simulink model "stellaris_lp_adc"  (R2017a)
settings: Solver=FixedStepDiscrete  StartTime=0.0  StopTime=10.0  FixedStep=0.2  RelTol=1e-3
libraries: stellaris_lp_lib x15, simulink x1
settings Model: ExtModeTrigDuration=2  Creator=peselnikmg  LastModifiedBy=Nilim
settings DataIOCC: LimitDataPoints=on  SaveFormat=Array  SignalLoggingSaveFormat=ModelDataLogs  ReturnWorkspaceOutputs=on
settings OptimizationCC: UseDivisionForNetSlopeComputation=on  UseFloatMulNetSlope=on  UseSpecifiedMinMax=on  PassReuseOutputArgsAs=Individual arguments  ExpressionDepthLimit=2147483647  ZeroExternalMemoryAtStartup=off  ZeroInternalMemoryAtStartup=off  NoFixptDivByZeroProtection=on  EfficientFloat2IntCast=on  LifeSpan=inf  MaxStackSize=64  OptimizeBlockOrder=speed
settings DebuggingCC: ReadBeforeWriteMsg=DisableAll  WriteAfterWriteMsg=DisableAll  WriteAfterReadMsg=DisableAll  MultiTaskDSMMsg=none  IntegerOverflowMsg=error  ParameterTunabilityLossMsg=error  AssertControl=DisableAll  StateNameClashWarn=warning  NonBusSignalsTreatedAsBus=error  SFInvalidInputDataAccessInChartInitDiag=error  SFTransitionOutsideNaturalParentDiag=error  SFUnreachableExecutionPathDiag=error  SFUndirectedBroadcastEventsDiag=error  SFExecutionAtInitializationDiag=none  IntegerSaturationMsg=error
settings HardwareCC: ProdBitPerPointer=32  ProdBitPerSizeT=32  ProdBitPerPtrDiffT=32  ProdLargestAtomicInteger=Long  ProdLargestAtomicFloat=Double  ProdWordSize=32  ProdHWDeviceType=ARM Compatible->ARM Cortex
settings ModelReferenceCC: UpdateModelReferenceTargets=IfOutOfDate  PropagateSignalLabelsOutOfModel=off
settings SFSimCC: SFSimEcho=off  MATLABDynamicMemAlloc=off
settings RTWCC: SystemTargetFile=ert.tlc  HardwareBoard=Tiva TM4C123G Launchpad  TLCOptions=-aInlineSetEventsForThisBaseRateFcn=TLC_FALSE -aSuppressMultiTaskScheduler=TLC_FALSE -aRateBasedStepFcn=1  TemplateMakefile=ert_default_tmf  Description=Embedded Coder  GenerateReport=on  RTWVerbose=off  Toolchain=Texas Instruments Code Composer Studio (Tiva)  IncludeHyperlinkInReport=on  LaunchReport=on  GenerateTraceInfo=on  GenerateTraceReport=on  GenerateTraceReportSl=on  GenerateTraceReportSf=on  GenerateTraceReportEml=on
settings CodeAppCC: ForceParamTrailComments=on  IgnoreCustomStorageClasses=off  OperatorAnnotations=on  SimulinkDataObjDesc=on  SFDataObjDesc=on  MATLABFcnDesc=on  CustomSymbolStrType=$N$R$M  InsertBlockDesc=on  MATLABSourceComments=on  EnableCustomComments=on  ReqsInCode=on
settings ERTTargetCC: UtilityFuncGeneration=Shared location  CombineSignalStateStructs=on  SuppressErrorStatus=on  SupportNonFinite=off  ParenthesesLevel=Maximum  CastingMode=Standards  EnableSignedLeftShifts=off  EnableSignedRightShifts=off
settings ConfigComp: CovMetricSettings=dw  CovHtmlReporting=on  CovSaveCumulativeToWorkspaceVar=on  CovSaveSingleToWorkspaceVar=on  CovExternalEMLEnable=off

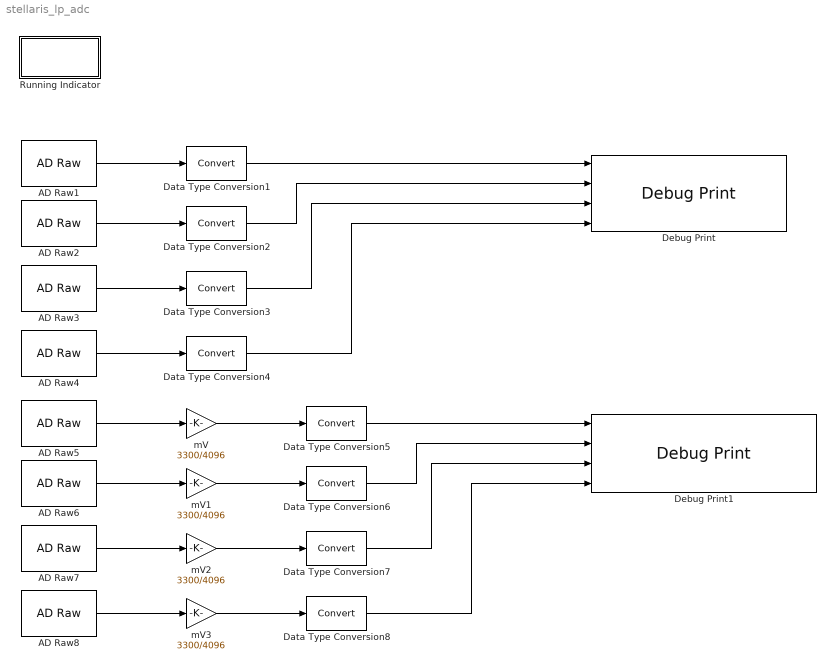
== system stellaris_lp_adc ==
  AD Raw1 : stellaris_lp_lib/ADC/AD Raw  ch="1   PE3"  sample_time=0.2
      settings: SourceProductName=Run on Stellaris LaunchPad
  AD Raw2 : stellaris_lp_lib/ADC/AD Raw  ch="2   PE2"  sample_time=0.2
      settings: SourceProductName=Run on Stellaris LaunchPad
  AD Raw3 : stellaris_lp_lib/ADC/AD Raw  ch="3   PE1"  sample_time=0.2
      settings: SourceProductName=Run on Stellaris LaunchPad
  AD Raw4 : stellaris_lp_lib/ADC/AD Raw  ch="4   PE0"  sample_time=0.2
      settings: SourceProductName=Run on Stellaris LaunchPad
  AD Raw5 : stellaris_lp_lib/ADC/AD Raw  ch="5   PE5"  sample_time=0.2
      settings: SourceProductName=Run on Stellaris LaunchPad
  AD Raw6 : stellaris_lp_lib/ADC/AD Raw  ch="6   PE4"  sample_time=0.2
      settings: SourceProductName=Run on Stellaris LaunchPad
  AD Raw7 : stellaris_lp_lib/ADC/AD Raw  ch="7   PB4"  sample_time=0.2
      settings: SourceProductName=Run on Stellaris LaunchPad
  AD Raw8 : stellaris_lp_lib/ADC/AD Raw  ch="8   PB5"  sample_time=0.2
      settings: SourceProductName=Run on Stellaris LaunchPad
  Data Type Conversion{1..8} (8 alike) : DataTypeConversion
  Debug Print : stellaris_lp_lib/Debug/Debug Print  fmt="'AD 1-4  = %d, %d, %d, %d'"  sample_time=-1
      settings: SourceProductName=Run on Stellaris LaunchPad
  Debug Print1 : stellaris_lp_lib/Debug/Debug Print  fmt="'AD 5-8  = %d, %d, %d, %d (unit mV)'"  sample_time=-1
      settings: SourceProductName=Run on Stellaris LaunchPad
  Running Indicator : Subsystem
  mV{,1..3} (4 alike) : Gain  Gain=3300/4096
  wires:
  Data Type Conversion1/1 -> Debug Print/1
  AD Raw1/1 -> Data Type Conversion1/1
  AD Raw2/1 -> Data Type Conversion2/1
  AD Raw3/1 -> Data Type Conversion3/1
  AD Raw4/1 -> Data Type Conversion4/1
  Data Type Conversion2/1 -> Debug Print/2
  Data Type Conversion3/1 -> Debug Print/3
  Data Type Conversion4/1 -> Debug Print/4
  Data Type Conversion5/1 -> Debug Print1/1
  AD Raw5/1 -> mV/1
  AD Raw6/1 -> mV1/1
  AD Raw7/1 -> mV2/1
  AD Raw8/1 -> mV3/1
  Data Type Conversion6/1 -> Debug Print1/2
  Data Type Conversion7/1 -> Debug Print1/3
  Data Type Conversion8/1 -> Debug Print1/4
  mV/1 -> Data Type Conversion5/1
  mV1/1 -> Data Type Conversion6/1
  mV2/1 -> Data Type Conversion7/1
  mV3/1 -> Data Type Conversion8/1

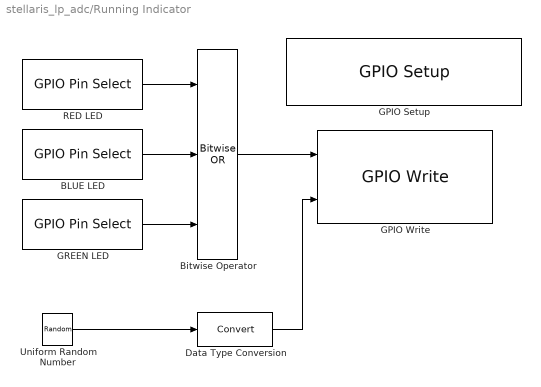
== system stellaris_lp_adc/Running Indicator ==
  BLUE LED : stellaris_lp_lib/GPIO/GPIO Pin Select  GPIO_PIN_X=GPIO_PIN_2
      settings: SourceProductName=Run on Stellaris LaunchPad
  Bitwise Operator : simulink/Logic and Bit Operations/Bitwise Operator  logicop=OR  UseBitMask=off  NumInputPorts=3  BitMask=bin2dec('11011001')  BitMaskRealWorld=Stored Integer
  Data Type Conversion : DataTypeConversion
  GPIO Setup : stellaris_lp_lib/GPIO/GPIO Setup  GPIO_PORTX_BASE=GPIO_PORTF_BASE  PinsOutput_0=Input  PinsOutput_1=Output  PinsOutput_2=Output  PinsOutput_3=Output  PinsOutput_4=Input  PinsOutput_5=Input  PinsOutput_6=Input  PinsOutput_7=Input
      settings: SourceProductName=Run on Stellaris LaunchPad
  GPIO Write : stellaris_lp_lib/GPIO/GPIO Write  GPIO_PORTX_BASE=GPIO_PORTF_BASE  SampleTime=-1
      settings: SourceProductName=Run on Stellaris LaunchPad
  GREEN LED : stellaris_lp_lib/GPIO/GPIO Pin Select  GPIO_PIN_X=GPIO_PIN_3
      settings: SourceProductName=Run on Stellaris LaunchPad
  RED LED : stellaris_lp_lib/GPIO/GPIO Pin Select  GPIO_PIN_X=GPIO_PIN_1
      settings: SourceProductName=Run on Stellaris LaunchPad
  Uniform Random Number : UniformRandomNumber  Minimum=2  Maximum=16  SampleTime=0.2
  wires:
  BLUE LED/1 -> Bitwise Operator/2
  RED LED/1 -> Bitwise Operator/1
  GREEN LED/1 -> Bitwise Operator/3
  Bitwise Operator/1 -> GPIO Write/1
  Uniform Random Number/1 -> Data Type Conversion/1
  Data Type Conversion/1 -> GPIO Write/2
